simulink model "circular_trajectory"  (R2023b)
settings: Solver=VariableStepAuto  StartTime=0.0  StopTime=10  RelTol=1e-3
libraries: uavutilslib x1
settings Model: Creator=rakshan  LastModifiedBy=rakshan

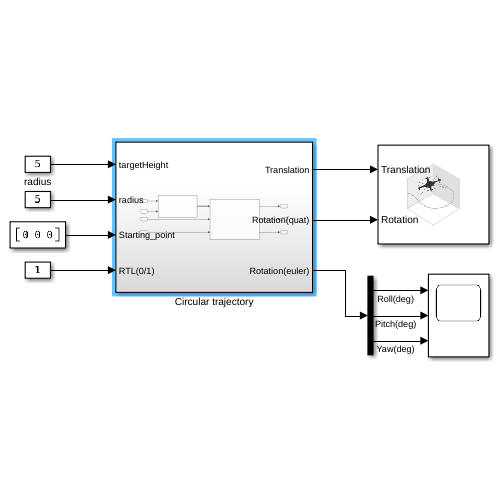
[thumbnail: Simulink's stored preview of the top-level diagram]
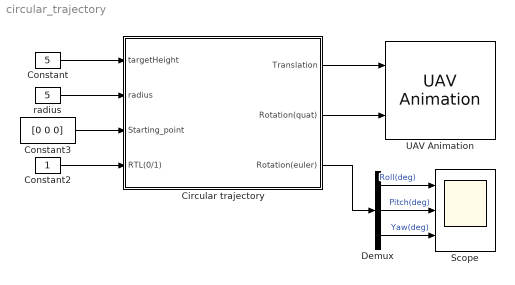
== system circular_trajectory ==
  Circular trajectory : Subsystem
  Constant : Constant  Value=5  OutDataTypeStr=double
  Constant2 : Constant
  Constant3 : Constant  Value=[0 0 0]  VectorParams1D=off
  Demux : Demux  Outputs=3
  Scope : Scope  NumInputPorts=3
  UAV Animation : uavutilslib/UAV Animation  UAVType=Multirotor  UAVSize=1  InertialZDirection=Up  SampleTime=-1
  radius : Constant  Value=5  OutDataTypeStr=double
  wires:
  Demux/1 -> Scope/1  "Roll(deg)"
  Demux/2 -> Scope/2  "Pitch(deg)"
  Demux/3 -> Scope/3  "Yaw(deg)"
  Constant/1 -> Circular trajectory/1(targetHeight)
  radius/1 -> Circular trajectory/2(radius)
  Constant3/1 -> Circular trajectory/3(Starting_point)
  Constant2/1 -> Circular trajectory/4(RTL(0/1))
  Circular trajectory/1(Translation) -> UAV Animation/1
  Circular trajectory/2(Rotation(quat)) -> UAV Animation/2
  Circular trajectory/3(Rotation(euler)) -> Demux/1

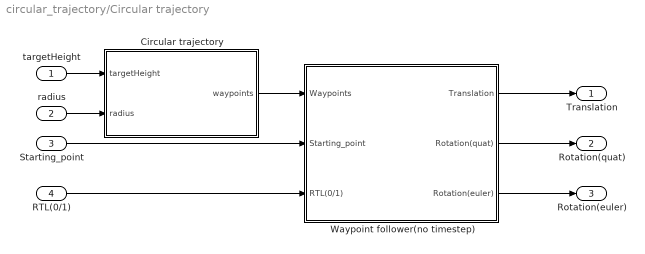
== system circular_trajectory/Circular trajectory ==
  targetHeight : Inport
  radius : Inport  Port=2
  Starting_point : Inport  Port=3
  RTL(0/1) : Inport  Port=4
  Circular trajectory : Subsystem
  Waypoint follower(no timestep) : Subsystem
  Translation : Outport
  Rotation(quat) : Outport  Port=2
  Rotation(euler) : Outport  Port=3
  wires:
  Waypoint follower(no timestep)/2(Rotation(quat)) -> Rotation(quat)/1
  radius/1 -> Circular trajectory/2(radius)
  RTL(0/1)/1 -> Waypoint follower(no timestep)/3(RTL(0/1))
  Waypoint follower(no timestep)/1(Translation) -> Translation/1
  targetHeight/1 -> Circular trajectory/1(targetHeight)
  Circular trajectory/1(waypoints) -> Waypoint follower(no timestep)/1(Waypoints)
  Waypoint follower(no timestep)/3(Rotation(euler)) -> Rotation(euler)/1
  Starting_point/1 -> Waypoint follower(no timestep)/2(Starting_point)

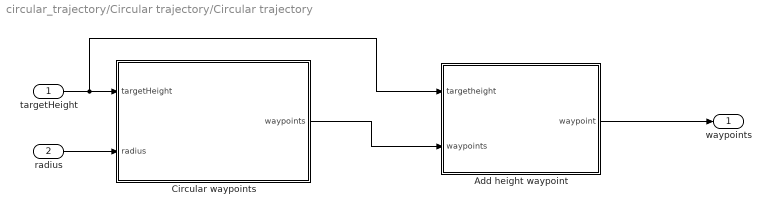
== system circular_trajectory/Circular trajectory/Circular trajectory ==
  targetHeight : Inport
  radius : Inport  Port=2
  Add height waypoint : MATLAB Function  TreatAsAtomicUnit=on
  Circular waypoints : MATLAB Function  TreatAsAtomicUnit=on
  waypoints : Outport
  wires:
  radius/1 -> Circular waypoints/2(radius)
  targetHeight/1 -> Add height waypoint/1(targetheight), Circular waypoints/1(targetHeight)
  Add height waypoint/1(waypoint) -> waypoints/1
  Circular waypoints/1(waypoints) -> Add height waypoint/2(waypoints)

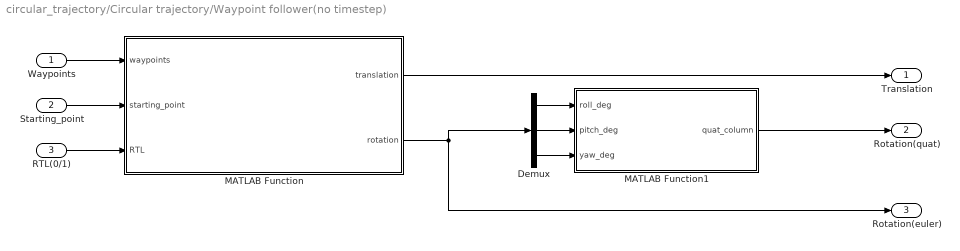
== system circular_trajectory/Circular trajectory/Waypoint follower(no timestep) ==
  Waypoints : Inport
  Starting_point : Inport  Port=2
  RTL(0/1) : Inport  Port=3
  Demux : Demux  Outputs=3
  MATLAB Function : MATLAB Function  TreatAsAtomicUnit=on
  MATLAB Function1 : MATLAB Function  TreatAsAtomicUnit=on
  Translation : Outport
  Rotation(quat) : Outport  Port=2
  Rotation(euler) : Outport  Port=3
  wires:
  Demux/1 -> MATLAB Function1/1(roll_deg)
  Demux/3 -> MATLAB Function1/3(yaw_deg)
  Demux/2 -> MATLAB Function1/2(pitch_deg)
  MATLAB Function1/1(quat_column) -> Rotation(quat)/1
  MATLAB Function/2(rotation) -> Demux/1, Rotation(euler)/1
  Waypoints/1 -> MATLAB Function/1(waypoints)
  Starting_point/1 -> MATLAB Function/2(starting_point)
  MATLAB Function/1(translation) -> Translation/1
  RTL(0/1)/1 -> MATLAB Function/3(RTL)

== matlab function circular_trajectory/Circular trajectory/Waypoint follower(no timestep)/MATLAB Function ==
  data: waypoints input; translation output; rotation output; starting_point input; RTL input
function [translation, rotation] = interpolateWaypointsSimulink(waypoints, starting_point, RTL)
    persistent current_waypoint current_index;

    % Concatenate waypoints for return-to-launch (RTL) if needed
    if RTL == 1
        waypoints = [starting_point; waypoints; starting_point];
    else
        waypoints = [starting_point; waypoints];
    end

    % Initialize persistent variables on the first call
    if isempty(current_waypoint)
        current_waypoint = waypoints(1, :);
        current_index = 1;
    end

    % Initialize outputs
    translation = zeros(1, 3);
    rotation = zeros(1, 3); % Euler angles: [yaw, pitch, roll]

    % Check if reached the last waypoint
    if current_index >= size(waypoints, 1)
        translation = waypoints(end, :);
        rotation = [0 0 0]; % No rotation (identity)
        return;
    end

    % Calculate the next waypoint
    next_waypoint = waypoints(current_index + 1, :);

    % Calculate the direction vector and step size
    direction_vector = next_waypoint - current_waypoint;
    distance_to_next_waypoint = norm(direction_vector);
    
    % Normalize direction vector if distance is greater than zero
    if distance_to_next_waypoint > 0
        direction_vector = direction_vector / distance_to_next_waypoint;
    end
    
    translation = next_waypoint;
    current_waypoint = next_waypoint;
    current_index = current_index + 1;
    

    % Calculate rotation angles (Euler angles)
    yaw = atan2(direction_vector(2), direction_vector(1));
    pitch = asin(direction_vector(3) / norm(direction_vector));
    roll = 0; % Assuming no roll motion

    % Update rotation
    rotation = [yaw, pitch, roll];
end

== matlab function circular_trajectory/Circular trajectory/Circular trajectory/Circular waypoints ==
  data: targetHeight input; waypoints output; radius input
function waypoints = generateWaypoints(targetHeight, radius)
% This function generates waypoints for a circular path around a target at a given height.

% Define the number of waypoints
numWaypoints = 30;

% Create an equally spaced angular vector
theta = linspace(0, 2*pi, numWaypoints);

waypoints = zeros(numWaypoints,3);
% Calculate waypoint positions in the XY plane
waypoints(:, 1) = radius * cos(theta);
waypoints(:, 2) = radius * sin(theta);

% Set the Z-coordinate of all waypoints to the target height
waypoints(:, 3) = targetHeight * ones(numWaypoints, 1);

end

== matlab function circular_trajectory/Circular trajectory/Waypoint follower(no timestep)/MATLAB Function1 ==
  data: roll_deg input; quat_column output; pitch_deg input; yaw_deg input
function quat_column = eulerToQuat(roll_deg, pitch_deg, yaw_deg)
    % Convert Euler angles to radians
    roll_rad = deg2rad(roll_deg);
    pitch_rad = deg2rad(pitch_deg);
    yaw_rad = deg2rad(yaw_deg);

    % Calculate half angles
    roll_half = roll_rad / 2;
    pitch_half = pitch_rad / 2;
    yaw_half = yaw_rad / 2;

    % Calculate trigonometric functions
    roll_sin = sin(roll_half);
    roll_cos = cos(roll_half);
    pitch_sin = sin(pitch_half);
    pitch_cos = cos(pitch_half);
    yaw_sin = sin(yaw_half);
    yaw_cos = cos(yaw_half);

    % Calculate quaternion components
    q0 = roll_cos * pitch_cos * yaw_cos + roll_sin * pitch_sin * yaw_sin;
    q1 = roll_sin * pitch_cos * yaw_cos - roll_cos * pitch_sin * yaw_sin;
    q2 = roll_cos * pitch_sin * yaw_cos + roll_sin * pitch_cos * yaw_sin;
    q3 = roll_cos * pitch_cos * yaw_sin - roll_sin * pitch_sin * yaw_cos;

    % Format the quaternion as a column vector
    quat_column = [q0; q1; q2; q3];
end

== matlab function circular_trajectory/Circular trajectory/Circular trajectory/Add height waypoint ==
  data: waypoint output; targetheight input; waypoints input
function waypoint = WayPoints(targetheight,waypoints)

waypoint1 = [0 0 targetheight];

waypoint = [waypoint1;waypoints];

end
